simulink model "simple_example"  (R2022a)
settings: Solver=ode4  StartTime=0.0  StopTime=20  FixedStep=step_size  MaxStep=1e-3  RelTol=1e-3  EnableMultiTasking=on
values from neighbouring files (symbols this model uses):
  Gamma = 1e8    (= 100000000)    [DoSim.m]
  k_sp = 1e3    (= 1000)    [DoSim.m]
  theta = 2    [DoSim.m]
libraries: vrlib x2
settings Model: Creator=li64  LastModifiedBy=Pan Zhao
settings SolverCC: AlgebraicLoopSolver=TrustRegion
settings DataIOCC: LimitDataPoints=on  SaveFormat=Array  SignalLoggingSaveFormat=ModelDataLogs  ReturnWorkspaceOutputs=off
settings OptimizationCC: ExpressionDepthLimit=2147483647  LifeSpan=inf
settings DebuggingCC: UnderspecifiedInitializationDetection=Classic  MergeDetectMultiDrivingBlocksExec=none  SolverPrmCheckMsg=warning  FcnCallInpInsideContextMsg=warning  UnconnectedInputMsg=warning  UnconnectedOutputMsg=warning  UnconnectedLineMsg=warning  StateNameClashWarn=warning  SFUnexpectedBacktrackingDiag=warning  SFNoUnconditionalDefaultTransitionDiag=warning  SFExecutionAtInitializationDiag=none  SFMachineParentedDataDiag=warning  ArithmeticOperatorsInVariantConditions=warning
settings HardwareCC: ProdBitPerPointer=32  ProdBitPerSizeT=32  ProdBitPerPtrDiffT=32  ProdLargestAtomicFloat=None  ProdIntDivRoundTo=Undefined  ProdEndianess=Unspecified  ProdWordSize=32  ProdHWDeviceType=32-bit Generic
settings ModelReferenceCC: PropagateSignalLabelsOutOfModel=off
settings SFSimCC: SimUseLocalCustomCode=off  CustomCodeUndefinedFunction=UseInterfaceOnly
settings RTWCC: RTWUseLocalCustomCode=off  DLArmComputeVersion=19.05
settings CodeAppCC: StateflowObjectComments=on
settings GRTTargetCC: TargetLangStandard=C89/C90 (ANSI)  CombineOutputUpdateFcns=off  GRTInterface=on
settings ConfigComp: CovMetricSettings=dw  CovSaveCumulativeToWorkspaceVar=on  CovSaveSingleToWorkspaceVar=on  CovExternalEMLEnable=off

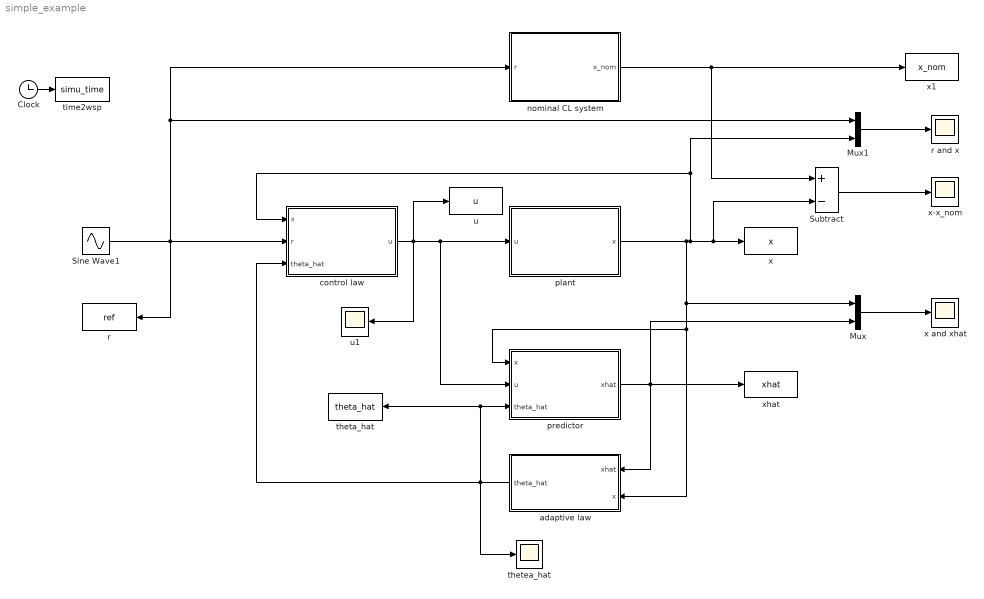
== system simple_example ==
  Clock : Clock
  Mux : Mux  Inputs=2
  Mux1 : Mux  Inputs=2
  Sine Wave1 : Sin  Amplitude=100  Frequency=0.5  SampleTime=0
  Subtract : Sum  Inputs=+-
  adaptive law : Subsystem
  control law : Subsystem
  nominal CL system : Subsystem
  plant : Subsystem
  predictor : Subsystem
  r : ToWorkspace  VariableName=ref  SampleTime=-1
  r and x : Scope
  theta_hat : ToWorkspace  VariableName=theta_hat  SampleTime=-1
  thetea_hat : Scope
  time2wsp : ToWorkspace  VariableName=simu_time  SampleTime=-1
  u : ToWorkspace  VariableName=u  SampleTime=-1
  u1 : Scope
  x : ToWorkspace  VariableName=x  SampleTime=-1
  x and xhat : Scope
  x-x_nom : Scope
  x1 : ToWorkspace  VariableName=x_nom  SampleTime=-1
  xhat : ToWorkspace  VariableName=xhat  SampleTime=-1
  wires:
  adaptive law/1(theta_hat) -> control law/3(theta_hat), thetea_hat/1, predictor/3(theta_hat), theta_hat/1
  control law/1(u) -> plant/1(u), predictor/2(u), u/1, u1/1
  predictor/1(xhat) -> Mux/2, xhat/1, adaptive law/1(xhat)
  Sine Wave1/1 -> control law/2(r), r/1, nominal CL system/1(r), Mux1/1
  Clock/1 -> time2wsp/1
  Mux/1 -> x and xhat/1
  Mux1/1 -> r and x/1
  nominal CL system/1(x_nom) -> Subtract/1, x1/1
  plant/1(x) -> Subtract/2, x/1, Mux1/2, control law/1(x), Mux/1, predictor/1(x), adaptive law/2(x)
  Subtract/1 -> x-x_nom/1

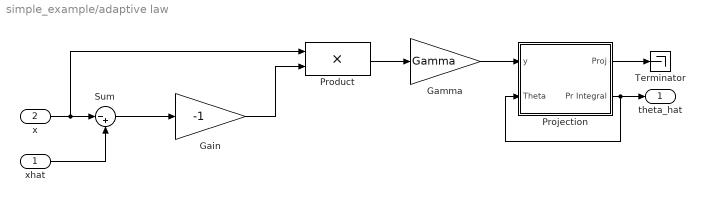
== system simple_example/adaptive law ==
  xhat : Inport
  x : Inport  Port=2
  Gain : Gain  Gain=-1
  Gamma : Gain  Gain=Gamma
  Product : Product  RndMeth=Zero
  Projection : Subsystem  mask{EpsilonTheta=0.3, Prmax=5, Pr0=0}
      mask prompts: EpsilonTheta "Epsilon"; Prmax "Bound (radius of the ball)"; Pr0 "Initialization of integral"
      mask help:
      | Computes projection of the signal and safely integrate it.
      | Works both for scalar and vector signals.
      | It considers the parameter set as a ball at the origin with setted radius.
      mask init:
      | Thetamax = Prmax / sqrt(EpsilonTheta+1);
  Sum : Sum  Inputs=|-+
  Terminator : Terminator
  theta_hat : Outport
  wires:
  Gamma/1 -> Projection/1(y)
  Product/1 -> Gamma/1
  Sum/1 -> Gain/1
  x/1 -> Sum/1, Product/1
  xhat/1 -> Sum/2
  Gain/1 -> Product/2
  Projection/2(Pr Integral) -> theta_hat/1, Projection/2(Theta)
  Projection/1(Proj) -> Terminator/1

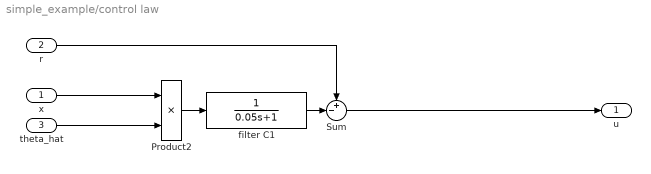
== system simple_example/control law ==
  x : Inport
  r : Inport  Port=2
  theta_hat : Inport  Port=3
  Product2 : Product  RndMeth=Zero
  Sum : Sum  Inputs=+-|
  filter C1 : TransferFcn  Denominator=[0.05 1]
  u : Outport
  wires:
  theta_hat/1 -> Product2/2
  r/1 -> Sum/1
  x/1 -> Product2/1
  Product2/1 -> filter C1/1
  Sum/1 -> u/1
  filter C1/1 -> Sum/2

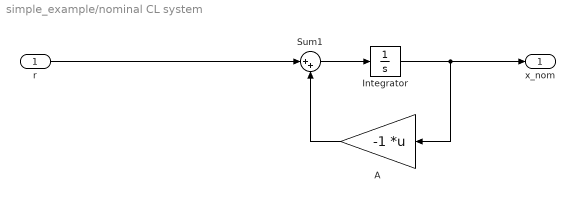
== system simple_example/nominal CL system ==
  r : Inport
  A : Gain  Gain=-1  Multiplication=Matrix(K*u)
  Integrator : Integrator
  Sum1 : Sum  Inputs=|++
  x_nom : Outport
  wires:
  r/1 -> Sum1/1
  Sum1/1 -> Integrator/1
  A/1 -> Sum1/2
  Integrator/1 -> A/1, x_nom/1

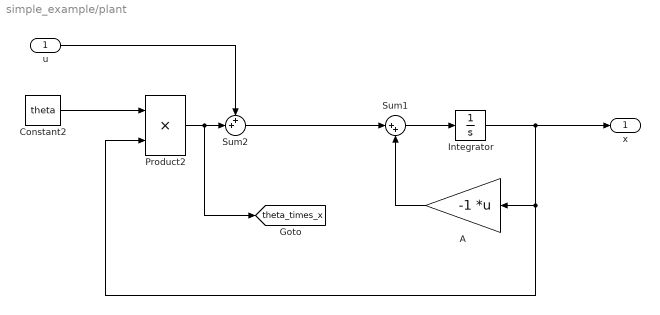
== system simple_example/plant ==
  u : Inport
  A : Gain  Gain=-1  Multiplication=Matrix(K*u)
  Constant2 : Constant  Value=theta
  Integrator : Integrator
  Product2 : Product  RndMeth=Zero
  Sum1 : Sum  Inputs=|++
  Sum2 : Sum  Inputs=++|
  x : Outport
  tag scope: theta_times_x=global
  wires:
  Integrator/1 -> x/1, A/1, Product2/2
  A/1 -> Sum1/2
  Sum1/1 -> Integrator/1
  Sum2/1 -> Sum1/1
  Constant2/1 -> Product2/1
  Product2/1 -> [theta_times_x], Sum2/2
  u/1 -> Sum2/1

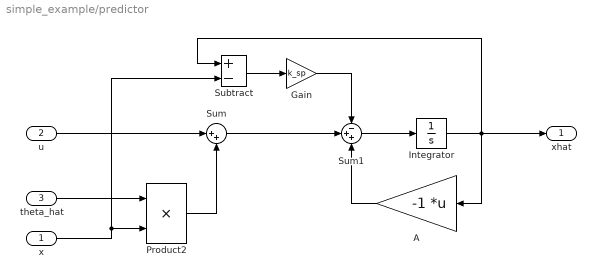
== system simple_example/predictor ==
  x : Inport
  u : Inport  Port=2
  theta_hat : Inport  Port=3
  A : Gain  Gain=-1  Multiplication=Matrix(K*u)
  Gain : Gain  Gain=k_sp
  Integrator : Integrator
  Product2 : Product  RndMeth=Zero
  Subtract : Sum  Inputs=+-
  Sum : Sum  Inputs=|++
  Sum1 : Sum  Inputs=-++
  xhat : Outport
  wires:
  u/1 -> Sum/1
  Product2/1 -> Sum/2
  Integrator/1 -> Subtract/1, A/1, xhat/1
  A/1 -> Sum1/3
  Sum1/1 -> Integrator/1
  Sum/1 -> Sum1/2
  theta_hat/1 -> Product2/1
  x/1 -> Subtract/2, Product2/2
  Subtract/1 -> Gain/1
  Gain/1 -> Sum1/1

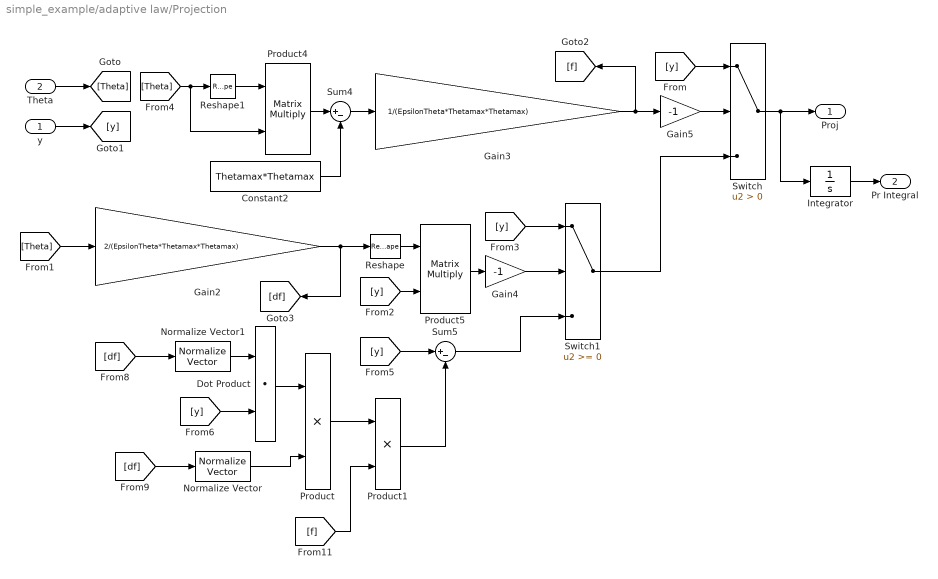
== system simple_example/adaptive law/Projection ==
  y : Inport
  Theta : Inport  Port=2
  Constant2 : Constant  Value=Thetamax*Thetamax
  Dot Product : DotProduct  OutDataTypeStr=Inherit: Inherit via internal rule
  Gain2 : Gain  Gain=2/(EpsilonTheta*Thetamax*Thetamax)
  Gain3 : Gain  Gain=1/(EpsilonTheta*Thetamax*Thetamax)
  Gain4 : Gain  Gain=-1
  Gain5 : Gain  Gain=-1
  Integrator : Integrator  InitialCondition=Pr0  LimitOutput=on  UpperSaturationLimit=Prmax  LowerSaturationLimit=-Prmax
  Normalize Vector : vrlib/Utilities/Normalize Vector  maxzero=0
  Normalize Vector1 : vrlib/Utilities/Normalize Vector  maxzero=0
  Product : Product  RndMeth=Zero
  Product1 : Product  RndMeth=Zero
  Product4 : Product  Multiplication=Matrix(*)  RndMeth=Zero
  Product5 : Product  Multiplication=Matrix(*)  RndMeth=Zero
  Reshape : Reshape  OutputDimensionality=Row vector (2-D)
  Reshape1 : Reshape  OutputDimensionality=Row vector (2-D)
  Sum4 : Sum  Inputs=|+-
  Sum5 : Sum  Inputs=|+-
  Switch : Switch  Criteria=u2 > Threshold  SaturateOnIntegerOverflow=off  InputSameDT=off
  Switch1 : Switch  SaturateOnIntegerOverflow=off  InputSameDT=off
  Proj : Outport
  Pr Integral : Outport  Port=2
  wires:
  Gain5/1 -> Switch/2
  Sum5/1 -> Switch1/3
  [y] -> Sum5/1
  Theta/1 -> [Theta]
  y/1 -> [y]
  Switch/1 -> Proj/1, Integrator/1
  Switch1/1 -> Switch/3
  [Theta] -> Gain2/1
  [y] -> Switch1/1
  Gain4/1 -> Switch1/2
  Product5/1 -> Gain4/1
  [y] -> Product5/2
  [y] -> Switch/1
  Gain3/1 -> [f], Gain5/1
  Sum4/1 -> Gain3/1
  Constant2/1 -> Sum4/2
  Product4/1 -> Sum4/1
  [Theta] -> Reshape1/1, Product4/2
  Gain2/1 -> Reshape/1, [df]
  Reshape/1 -> Product5/1
  Reshape1/1 -> Product4/1
  [df] -> Normalize Vector1/1
  [df] -> Normalize Vector/1
  Normalize Vector1/1 -> Dot Product/1
  [y] -> Dot Product/2
  Dot Product/1 -> Product/1
  Normalize Vector/1 -> Product/2
  Product/1 -> Product1/1
  [f] -> Product1/2
  Product1/1 -> Sum5/2
  Integrator/1 -> Pr Integral/1
